simulink library "microgridLibrary"  (R2019b)
settings: Solver=VariableStepAuto  StartTime=0.0  StopTime=10.0  RelTol=1e-3
undefined symbols (not defined in the file or in its folder): Aa, BR, D1, Delta, DiscIntNeverNeededParam, Fn, gcbh, Ion, kv, Lithium, Ls, Pa, Pb, Pc, Rs, sps_rtmsupport, StationData, Ts, Ts_Control, Vn, Vnom
libraries: powerlib x80, simulink x29, powerlib_meascontrol x28, sps_avr x5, spsDieselMotorModel x3, electricdrivelib x2, re_lib x1
(part 3 of 6)

== system microgridLibrary/Diesel Generator (GOV, AVR only)/Selected Measurements ==
  m : Inport
  Bus Creator : BusCreator  Inputs=7
  Bus Selector : BusSelector  OutputSignals="Mechanical.Electrical power  Pe (pu),Mechanical.Rotor speed  wm  (pu),Output active power   Peo (pu),Output reactive power  Qeo (pu)"
  to W : Gain  Gain=Pn
  to W1 : Gain  Gain=Pn
  to W2 : Gain  Gain=Pn
  sm : Outport  VectorParamsAs1DForOutWhenUnconnected=off
  wires:
  to W2/1 -> Bus Creator/7  "Reactive Power (W)"
  to W1/1 -> Bus Creator/6  "Active Power (W)"
  Bus Selector/2 -> Bus Creator/3  "<Rotor speed  wm  (pu)>"
  Bus Creator/1 -> sm/1
  to W/1 -> Bus Creator/1  "Electrical Power (W)"
  Bus Selector/3 -> Bus Creator/4, to W1/1  "<Output active power   Peo (pu)>"
  Bus Selector/1 -> to W/1, Bus Creator/2  "<Electrical power  Pe (pu)>"
  Bus Selector/4 -> Bus Creator/5, to W2/1  "<Output reactive power  Qeo (pu)>"
  m/1 -> Bus Selector/1

== system microgridLibrary/Diesel Generator (Simple Controls)/Continuous ==
  wref (pu) : Inport
  Vref (pu) : Inport  Port=2
  Diesel Engine Governor : spsDieselMotorModel/Diesel Engine Governor  K=29  Tr=[0.01 0.02 0.2]  Ta=[0.25 0.009 0.0384]  Tlim=[0 1.1]  Td=0.024  Pm0=0.84379
      settings: SourceProductName=Simscape Electrical  SourceProductBaseCode=PS
  Excitation System : sps_avr/AC1A Excitation System  Tr=20e-3  KaTa=[400 0.02]  VAminmax=[-14.5 14.5]  VRminmax=[-5.43 6.03]  KfTf=[0.03 1.0]  TbTc=[0 0]  KeTe=[1.0 0.80]  Ve12=[4.18 3.14]  SeVe12=[0.10 0.03]  Kd=0.38  Kc=0.20  v0=[1 1.3376]  TsBlock=0
      settings: SourceProductName=Simscape Electrical  SourceProductBaseCode=PS
  Generator Measures : Subsystem
  Ground : Ground
  Selected Measurements : Subsystem
  Shunt : powerlib/Elements/Three-Phase Parallel RLC Load  LConnTagsString=A|B|C  Configuration=Y (grounded)  NominalVoltage=Vn  Vabc=[1e3 1e3 1e3]  Vabcp=[1e3 1e3 1e3]  NominalFrequency=Fn  UnbalancedPower=off  ActivePower=Pn*0.05  InductivePower=0  CapacitivePower=0  Pabc=[10e3 9e3 11e3]  QLabc=[100 90 110]  QCabc=[100 90 110]  Pabcp=[10e3 9e3 11e3]  QLabcp=[100 90 110]  QCabcp=[100 90 110]  Measurements=None  LoadType=constant Z
      settings: SourceProductName=Simscape Electrical
  Synchronous Machine : powerlib/Machines/Synchronous Machine pu Standard  PresetModel=No  MechanicalLoad=Mechanical power Pm  ShowDetailedParameters=on  RotorType=Salient-pole  Units=per unit standard parameters  MeasurementBus=off  NominalParameters=[ Pn Vn Fn]  Reactances1=[ 1.81, 0.3, 0.23, 1.76, 0.65, 0.25, 0.15 ]  Reactances2="[ 1.305, 0.296, 0.252, 0.474,  0.243,  0.18 ]"  dAxisTimeConstants=Open-circuit  qAxisTimeConstants=Short-circuit  TimeConstants1="[ 4.4849  0.0681  0.1  ]"  TimeConstants2=[ 8.0, 0.03, 1.0, 0.07 ]  TimeConstants3="[  4.49  0.0681  0.0513  ]"  TimeConstants4=[ 8.0, 0.03, 0.3371, 0.0295 ]  TimeConstants5=[ 1.01, 0.053, 0.1 ]  TimeConstants6=[ 1.3201, 0.023, 1.0, 0.07 ]  TimeConstants7=[0.012 0.003 0.003]  TimeConstants8=[ 1.3201, 0.0231, 0.3371, 0.0295 ]  StatorResistance=0.003  Mechanical=[3.7 0 1 ]  PolePairs=20  InitialConditions=[0 -68.3001 0.841667 0.841667 0.841667 4.44859e-14 -120 120 1.3376]  SetSaturation=off  Saturation=[0.6404,0.7127,0.8441,0.9214,0.9956,1.082,1.19,1.316,1.457;0.7,0.7698,0.8872,0.9466,0.9969,1.046,1.1,1.151,1.201]  LoadFlowParameters=[1,0,0,0,0]  TsPowergui=0  TsBlock=-1  IterativeModel=Trapezoidal non iterative  IterativeDiscreteModel=Trapezoidal non iterative  BusType=swing  Pref=Pn*P0  Qref=0  Qmin=-inf  Qmax=inf  PLF=0  QLF=0
      settings: SourceProductName=Simscape Electrical
  A : PMIOPort  Side=Right
  B : PMIOPort  Port=2  Side=Right
  C : PMIOPort  Port=3  Side=Right
  m : Outport  VectorParamsAs1DForOutWhenUnconnected=off
  wires:
  Generator Measures/3(wm) -> Diesel Engine Governor/2
  Vref (pu)/1 -> Excitation System/1
  Selected Measurements/1(sm) -> m/1
  Synchronous Machine/1 -> Generator Measures/1(m), Selected Measurements/1(m)
  Ground/1 -> Excitation System/4
  Generator Measures/1(Ifd) -> Excitation System/3
  Diesel Engine Governor/1 -> Synchronous Machine/1
  wref (pu)/1 -> Diesel Engine Governor/1
  Excitation System/1 -> Synchronous Machine/2
  Generator Measures/2(Vt) -> Excitation System/2
  connections:
  Synchronous Machine/RConn1 -- Shunt/LConn1 -- A/RConn1
  Synchronous Machine/RConn3 -- Shunt/LConn3 -- C/RConn1
  Synchronous Machine/RConn2 -- Shunt/LConn2 -- B/RConn1

== system microgridLibrary/Diesel Generator (Simple Controls)/Discrete ==
  wref (pu) : Inport
  Vref (pu) : Inport  Port=2
  Diesel Engine Governor : Subsystem  mask(Diesel Engine & Governor){K=29, Tr=[0.01 0.02 0.2], Ta=[0.25 0.009 0.0384], Tlim=[0 1.1], Td=0.024, Pm0=0.84379, Ts=Ts}
      mask prompts: K "Regulator gain K:"; Tr "Regulator time constants [T1 T2 T3 ] (s) :"; Ta "Actuator time constants [T4 T5 T6] (s) :"; Tlim "Torque limits [Tmin Tmax] (pu) :"; Td "Engine time delay Td (s) :"; Pm0 "Initial value of mechanical power  Pm0 (pu) :"; Ts "Sample Time (s)"
      mask help:
      | This block implements a diesel engine and governor system:
      | 1st and 2nd inputs: Desired and actual speed (pu)
      | Output: Diesel engine mechanical power.Motor inertia should be combined with generator.
      | Controller transfer function:
      |      Hc=K.(1+T3.s)/(1+T1.s+T1.T2.s^2)
      | Actuator transfer function :
      |      Ha= (1+T4.s) / [ (s (1+T5.s)(1+T6.s) ]
      | Motor :
      |      Time delay Td
      |
      | (See reference in Tutorial Session 5)
  Excitation System : sps_avr/AC1A Excitation System  Tr=20e-3  KaTa=[400 0.02]  VAminmax=[-14.5 14.5]  VRminmax=[-5.43 6.03]  KfTf=[0.03 1.0]  TbTc=[0 0]  KeTe=[1.0 0.80]  Ve12=[4.18 3.14]  SeVe12=[0.10 0.03]  Kd=0.38  Kc=0.20  v0=[1 1.3376]  TsBlock=Ts
      settings: SourceProductName=Simscape Electrical  SourceProductBaseCode=PS
  Generator Measures : Subsystem
  Ground : Ground
  Selected Measurements : Subsystem
  Shunt : powerlib/Elements/Three-Phase Parallel RLC Load  LConnTagsString=A|B|C  Configuration=Y (grounded)  NominalVoltage=Vn  Vabc=[1e3 1e3 1e3]  Vabcp=[1e3 1e3 1e3]  NominalFrequency=Fn  UnbalancedPower=off  ActivePower=Pn*0.05  InductivePower=0  CapacitivePower=0  Pabc=[10e3 9e3 11e3]  QLabc=[100 90 110]  QCabc=[100 90 110]  Pabcp=[10e3 9e3 11e3]  QLabcp=[100 90 110]  QCabcp=[100 90 110]  Measurements=None  LoadType=constant Z
      settings: SourceProductName=Simscape Electrical
  Synchronous Machine : powerlib/Machines/Synchronous Machine pu Standard  PresetModel=No  MechanicalLoad=Mechanical power Pm  ShowDetailedParameters=on  RotorType=Salient-pole  Units=per unit standard parameters  MeasurementBus=off  NominalParameters=[ Pn Vn Fn]  Reactances1=[ 1.81, 0.3, 0.23, 1.76, 0.65, 0.25, 0.15 ]  Reactances2="[ 1.305, 0.296, 0.252, 0.474,  0.243,  0.18 ]"  dAxisTimeConstants=Open-circuit  qAxisTimeConstants=Short-circuit  TimeConstants1="[ 4.4849  0.0681  0.1  ]"  TimeConstants2=[ 8.0, 0.03, 1.0, 0.07 ]  TimeConstants3="[  4.49  0.0681  0.0513  ]"  TimeConstants4=[ 8.0, 0.03, 0.3371, 0.0295 ]  TimeConstants5=[ 1.01, 0.053, 0.1 ]  TimeConstants6=[ 1.3201, 0.023, 1.0, 0.07 ]  TimeConstants7=[0.012 0.003 0.003]  TimeConstants8=[ 1.3201, 0.0231, 0.3371, 0.0295 ]  StatorResistance=0.003  Mechanical=[3.7 0 1 ]  PolePairs=20  InitialConditions=[0 -68.3001 0.841667 0.841667 0.841667 4.44859e-14 -120 120 1.3376]  SetSaturation=off  Saturation=[0.6404,0.7127,0.8441,0.9214,0.9956,1.082,1.19,1.316,1.457;0.7,0.7698,0.8872,0.9466,0.9969,1.046,1.1,1.151,1.201]  LoadFlowParameters=[1,0,0,0,0]  TsPowergui=0  TsBlock=Ts  IterativeModel=Trapezoidal non iterative  IterativeDiscreteModel=Trapezoidal non iterative  BusType=PQ  Pref=Pn*P0  Qref=0  Qmin=-inf  Qmax=inf  PLF=0  QLF=0
      settings: SourceProductName=Simscape Electrical
  A : PMIOPort  Side=Right
  B : PMIOPort  Port=2  Side=Right
  C : PMIOPort  Port=3  Side=Right
  m : Outport  VectorParamsAs1DForOutWhenUnconnected=off
  wires:
  Excitation System/1 -> Synchronous Machine/2
  wref (pu)/1 -> Diesel Engine Governor/1(wref (pu))
  Diesel Engine Governor/1(Pmec (pu)) -> Synchronous Machine/1
  Generator Measures/1(Ifd) -> Excitation System/3
  Ground/1 -> Excitation System/4
  Synchronous Machine/1 -> Selected Measurements/1(m), Generator Measures/1(m)
  Selected Measurements/1(sm) -> m/1
  Generator Measures/2(Vt) -> Excitation System/2
  Vref (pu)/1 -> Excitation System/1
  Generator Measures/3(wm) -> Diesel Engine Governor/2(w (pu))
  connections:
  Synchronous Machine/RConn2 -- Shunt/LConn2 -- B/RConn1
  Synchronous Machine/RConn3 -- Shunt/LConn3 -- C/RConn1
  Synchronous Machine/RConn1 -- Shunt/LConn1 -- A/RConn1

== system microgridLibrary/Energy Storage (PQ Model)/Charge Limits ==
  SOC (%) : Inport
  Pin : Inport  Port=2
  Qin : Inport  Port=3
  Overcharge Check : Subsystem
  Undercharge Check : Subsystem
  Pbatt : Outport  VectorParamsAs1DForOutWhenUnconnected=off
  Qbatt : Outport  Port=2  VectorParamsAs1DForOutWhenUnconnected=off
  wires:
  SOC (%)/1 -> Overcharge Check/1(SOC (%)), Undercharge Check/1(SOC (%))
  Undercharge Check/2(Qout) -> Qbatt/1
  Pin/1 -> Overcharge Check/2(Pin)
  Overcharge Check/1(Pout) -> Undercharge Check/2(Pin)
  Qin/1 -> Overcharge Check/3(Qin)
  Undercharge Check/1(Pout) -> Pbatt/1  "Pbatt"
  Overcharge Check/2(Qout) -> Undercharge Check/3(Qin)

== system microgridLibrary/Energy Storage (PQ Model)/Disable PQ Source if VF Control ==
  Pdes : Inport
  Mode : Inport  Port=2
  Qdes : Inport  Port=3
  Constant : Constant  Value=0
  Constant1 : Constant  Value=0
  Switch2 : Switch  Criteria=u2 > Threshold
  Switch3 : Switch  Criteria=u2 > Threshold
  Pbatt : Outport  VectorParamsAs1DForOutWhenUnconnected=off
  Qbatt : Outport  Port=2  VectorParamsAs1DForOutWhenUnconnected=off
  wires:
  Mode/1 -> Switch3/2, Switch2/2
  Pdes/1 -> Switch2/1
  Switch2/1 -> Pbatt/1
  Constant1/1 -> Switch3/3
  Switch3/1 -> Qbatt/1
  Constant/1 -> Switch2/3
  Qdes/1 -> Switch3/1

== system microgridLibrary/Energy Storage (PQ Model)/Power Measures ==
  EMT : Subsystem  VariantControl=EMT
  Phasor : Subsystem  VariantControl=Phasor
  A : PMIOPort  Side=Left
  a : PMIOPort  Port=2  Side=Right
  B : PMIOPort  Port=3  Side=Left
  b : PMIOPort  Port=4  Side=Right
  C : PMIOPort  Port=5  Side=Left
  c : PMIOPort  Port=6  Side=Right
  P : Outport  VectorParamsAs1DForOutWhenUnconnected=off
  Q : Outport  Port=2  VectorParamsAs1DForOutWhenUnconnected=off

== system microgridLibrary/Energy Storage (PQ Model)/Reactive Power Capability ==
  Pin : Inport
  Qin : Inport  Port=2
  Constant : Constant  Value=Pnom
  Math Function : Math  Operator=square  SaturateOnIntegerOverflow=on
  Math Function1 : Math  Operator=square  SaturateOnIntegerOverflow=on
  Saturation Dynamic : simulink/Discontinuities/Saturation Dynamic  OutMin=[]  OutMax=[]  OutDataTypeStr=Inherit: Same as second input  OutDataType=fixdt(1, 16)  OutScaling=2^-10  DoSatur=off
  Sqrt : Sqrt  SaturateOnIntegerOverflow=on
  Sum : Sum  Inputs=-+|
  Unary Minus : UnaryMinus
  Qout : Outport  VectorParamsAs1DForOutWhenUnconnected=off
  wires:
  Sqrt/1 -> Saturation Dynamic/1, Unary Minus/1
  Math Function1/1 -> Sum/1
  Math Function/1 -> Sum/2
  Constant/1 -> Math Function/1
  Sum/1 -> Sqrt/1
  Unary Minus/1 -> Saturation Dynamic/3
  Saturation Dynamic/1 -> Qout/1
  Pin/1 -> Math Function1/1
  Qin/1 -> Saturation Dynamic/2

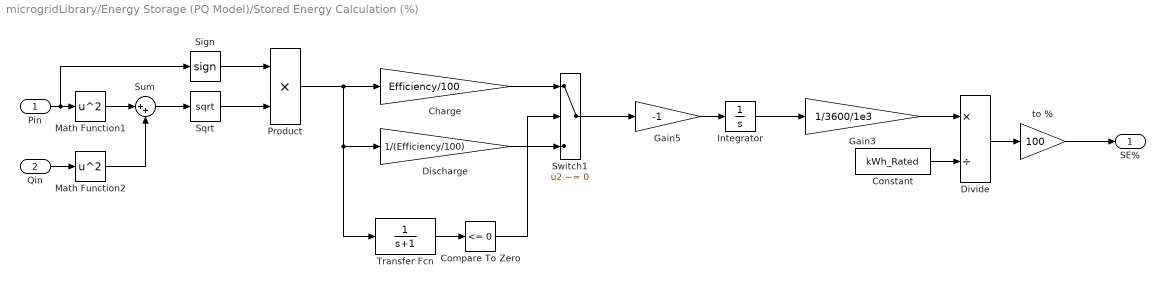
== system microgridLibrary/Energy Storage (PQ Model)/Stored Energy Calculation (%) ==
  Pin : Inport
  Qin : Inport  Port=2
  Charge : Gain  Gain=Efficiency/100
  Compare To Zero : simulink/Logic and Bit Operations/Compare To Zero  relop=<=  OutDataTypeStr=boolean
  Constant : Constant  Value=kWh_Rated
  Discharge : Gain  Gain=1/(Efficiency/100)
  Divide : Product  Inputs=*/
  Gain3 : Gain  Gain=1/3600/1e3
  Gain5 : Gain  Gain=-1
  Integrator : Integrator  InitialCondition=(Initial_kWh_pc/100)*kWh_Rated*3600*1e3
  Math Function1 : Math  Operator=square  SaturateOnIntegerOverflow=on
  Math Function2 : Math  Operator=square  SaturateOnIntegerOverflow=on
  Product : Product
  Sign : Signum
  Sqrt : Sqrt  SaturateOnIntegerOverflow=on
  Sum : Sum  Inputs=|++
  Switch1 : Switch  Criteria=u2 ~= 0
  Transfer Fcn : TransferFcn  Denominator=[1 1]
  to % : Gain  Gain=100
  SE% : Outport  VectorParamsAs1DForOutWhenUnconnected=off
  wires:
  Sign/1 -> Product/1
  Sqrt/1 -> Product/2
  Sum/1 -> Sqrt/1
  Math Function2/1 -> Sum/2
  Math Function1/1 -> Sum/1
  Qin/1 -> Math Function2/1
  Pin/1 -> Math Function1/1, Sign/1
  Product/1 -> Transfer Fcn/1, Discharge/1, Charge/1
  Discharge/1 -> Switch1/3
  Gain5/1 -> Integrator/1
  to %/1 -> SE%/1
  Transfer Fcn/1 -> Compare To Zero/1
  Switch1/1 -> Gain5/1
  Gain3/1 -> Divide/1
  Constant/1 -> Divide/2
  Charge/1 -> Switch1/1
  Divide/1 -> to %/1
  Compare To Zero/1 -> Switch1/2
  Integrator/1 -> Gain3/1

== system microgridLibrary/Fault /Fault A ==
  c : Inport
  Breaker : PMComponent  PhysicalDomain=powersysdomain  LeftPortType=p1  RightPortType=p1  LConnTagsString=a  RConnTagsString=__new0  mask(InnerPowersysBlock){}
  ITAIL : Terminator
  Model : Subsystem
  1 : PMIOPort  Side=Left
  2 : PMIOPort  Port=2  Side=Right
  tag scope: LibraryTag=global
  wires:
  [LibraryTag] -> ITAIL/1
  Model/1(gate) -> [LibraryTag]
  [LibraryTag] -> Model/2(Uswitch)
  c/1 -> Model/1("gate ")
  connections:
  1/RConn1 -- Breaker/LConn1
  2/RConn1 -- Breaker/RConn1

== system microgridLibrary/Fault /Fault B ==
  c : Inport
  Breaker : PMComponent  PhysicalDomain=powersysdomain  LeftPortType=p1  RightPortType=p1  LConnTagsString=a  RConnTagsString=__new0  mask(InnerPowersysBlock){}
  ITAIL : Terminator
  Model : Subsystem
  1 : PMIOPort  Side=Left
  2 : PMIOPort  Port=2  Side=Right
  tag scope: LibraryTag=global
  wires:
  [LibraryTag] -> ITAIL/1
  Model/1(gate) -> [LibraryTag]
  [LibraryTag] -> Model/2(Uswitch)
  c/1 -> Model/1("gate ")
  connections:
  1/RConn1 -- Breaker/LConn1
  2/RConn1 -- Breaker/RConn1

== system microgridLibrary/Fault /Fault C ==
  c : Inport
  Breaker : PMComponent  PhysicalDomain=powersysdomain  LeftPortType=p1  RightPortType=p1  LConnTagsString=a  RConnTagsString=__new0  mask(InnerPowersysBlock){}
  ITAIL : Terminator
  Model : Subsystem
  1 : PMIOPort  Side=Left
  2 : PMIOPort  Port=2  Side=Right
  tag scope: LibraryTag=global
  wires:
  [LibraryTag] -> ITAIL/1
  Model/1(gate) -> [LibraryTag]
  [LibraryTag] -> Model/2(Uswitch)
  c/1 -> Model/1("gate ")
  connections:
  1/RConn1 -- Breaker/LConn1
  2/RConn1 -- Breaker/RConn1

== system microgridLibrary/Grid Source Phasor Load Flow/Model ==
  Constant : Constant  Value=complex(cos(Pa),sin(Pa))
  Constant1 : Constant  Value=complex(cos(Pb),sin(Pb))
  Constant2 : Constant  Value=complex(cos(Pc),sin(Pc))
  Gain : Gain  Gain=Aa
  Initial Voltage : Subsystem
  Mux : Mux  Inputs=3
  Product : Product
  Out1 : Outport
  wires:
  Constant1/1 -> Mux/2
  Constant/1 -> Mux/1
  Constant2/1 -> Mux/3
  Mux/1 -> Product/1
  Product/1 -> Out1/1
  Initial Voltage/1(Aa) -> Gain/1
  Gain/1 -> Product/2

== system microgridLibrary/Grid-Connected Battery (EMT with Simple Controls)/Battery Controller ==
  m : Inport
  PQref : Inport  Port=2
  Compute PQ : Subsystem
  "P,Q Control " : Subsystem  TreatAsAtomicUnit=on
  to PU : Gain  Gain=1/Pnom
  Idq_ref : Outport  VectorParamsAs1DForOutWhenUnconnected=off
  wires:
  "P,Q Control "/1(Idq_ref) -> Idq_ref/1
  to PU/1 -> "P,Q Control "/1(PQref)
  m/1 -> Compute PQ/1(m)
  PQref/1 -> to PU/1
  Compute PQ/1(PQm) -> "P,Q Control "/2(m)

== system microgridLibrary/Grid-Connected Battery (EMT with Simple Controls)/DC Link ==
  C1 : powerlib/Elements/Series RLC Branch  LConnTagsString=__new0  RConnTagsString=__new0  BranchType=C  Resistance=1.0  Inductance=1.0  SetiL0=off  InitialCurrent=0  Capacitance=Clink  Setx0=on  InitialVoltage=Vnom_dc/2  Measurements=None
      settings: SourceProductName=Simscape Electrical
  C2 : powerlib/Elements/Series RLC Branch  LConnTagsString=__new0  RConnTagsString=__new0  BranchType=C  Resistance=1e5  Inductance=1.0  SetiL0=off  InitialCurrent=0  Capacitance=Clink  Setx0=on  InitialVoltage=Vnom_dc/2  Measurements=None
      settings: SourceProductName=Simscape Electrical
  PV+ : PMIOPort  Side=Left
  PV-- : PMIOPort  Port=2  Side=Left
  Inv+ : PMIOPort  Port=3  Side=Right
  N : PMIOPort  Port=4  Side=Right
  Inv-- : PMIOPort  Port=5  Side=Right
  connections:
  Inv--/RConn1 -- PV--/RConn1 -- C2/RConn1
  C1/RConn1 -- N/RConn1 -- C2/LConn1
  Inv+/RConn1 -- PV+/RConn1 -- C1/LConn1

== system microgridLibrary/Grid-Connected Battery (EMT with Simple Controls)/Grid Inverter ==
  note: Harmonic Filter
  Uref : Inport
  10 kvar : powerlib/Elements/Three-Phase Series RLC Load  LConnTagsString=A|B|C  Configuration=Delta  NominalVoltage=Vnom_sec  Vabc=[1e3 1e3 1e3]  Vabcp=[1e3 1e3 1e3]  NominalFrequency=Fnom  UnbalancedPower=off  ActivePower=Pc  InductivePower=0  CapacitivePower=Qc  Pabc=[10e3 9e3 11e3]  QLabc=[100 90 110]  QCabc=[100 90 110]  Pabcp=[10e3 9e3 11e3]  QLabcp=[100 90 110]  QCabcp=[100 90 110]  Measurements=None  LoadType=constant Z
      settings: SourceProductName=Simscape Electrical
  100 kVA 260V / 25 kV : powerlib/Elements/Three-Phase Transformer (Two Windings)  Winding1Connection=Yg  Winding2Connection=Delta (D1)  CoreType=Three single-phase transformers  SetSaturation=off  Hysteresis=off  DataFile='hysteresis'  SetInitialFlux=off  Measurements=None  UNITS=pu  NominalPower=[Pnom Fnom ]  Winding1=[ Vnom_prim , Rxf/2 , Lxf/2 ]  Winding2=[ Vnom_sec , Rxf/2 , Lxf/2 ]  Rm=200  Lm=200  L0=0.5  Saturation=[ 0,0 ; 0.0024,1.2 ; 1.0,1.52 ]  InitialFluxes=[ 0.8 , -0.8 , 0.7 ]  BreakLoop=off  DiscreteSolver=Trapezoidal iterative  DataType=off  TransfoNumber=0
      settings: SourceProductName=Simscape Electrical
  B1 : powerlib/Measurements/Three-Phase V-I Measurement  VoltageMeasurement=phase-to-ground  SetLabelV=off  LabelV=Vabc_B1  Vpu=off  VpuLL=off  CurrentMeasurement=yes  SetLabelI=off  LabelI=Iabc_B1  Ipu=off  Pbase=100e6  Vbase=500e3  OutputType=Magnitude  PhasorSimulation=off  PSBequivalent=0
      settings: SourceProductName=Simscape Electrical
  Bus Creator : BusCreator  Inputs=2
  Ground : Ground
  L : powerlib/Elements/Three-Phase Series RLC Branch  LConnTagsString=A|B|C  RConnTagsString=A|B|C  BranchType=RL  Resistance=Rchoke*Zbase  Inductance=Lchoke*Zbase/(2*pi*Fnom)  Capacitance=inf  Measurements=None
      settings: SourceProductName=Simscape Electrical
  Three-Level NPC Converter : powerlib/Power Electronics/Three-Level NPC Converter  ModelType=Average model (Uref-controlled)  Ron=1e-3  Rs=1e6  Cs=inf  Vforward=[0,0]  Ron_Diode=1e-3  Rs_Diode=1e6  Cs_Diode=inf  Vf_Diode=1e-3  Rs_CurrentSource=inf
      settings: SourceProductName=Simscape Electrical  SourceProductBaseCode=PS
  Inv+ : PMIOPort  Side=Left
  N : PMIOPort  Port=2  Side=Left
  Inv-- : PMIOPort  Port=3  Side=Left
  A : PMIOPort  Port=4  Side=Right
  B : PMIOPort  Port=5  Side=Right
  C : PMIOPort  Port=6  Side=Right
  m : Outport  VectorParamsAs1DForOutWhenUnconnected=off
  wires:
  Uref/1 -> Three-Level NPC Converter/1
  B1/1 -> Bus Creator/1  "Vabc"
  B1/2 -> Bus Creator/2  "Iabc"
  Bus Creator/1 -> m/1
  Ground/1 -> Three-Level NPC Converter/2
  connections:
  B1/RConn3 -- C/RConn1
  B1/RConn2 -- B/RConn1
  B1/RConn1 -- A/RConn1
  10 kvar/LConn1 -- 100 kVA 260V / 25 kV/RConn1 -- L/RConn1
  Three-Level NPC Converter/RConn1 -- Inv+/RConn1
  Three-Level NPC Converter/RConn3 -- Inv--/RConn1
  L/RConn3 -- 100 kVA 260V / 25 kV/RConn3 -- 10 kvar/LConn3
  L/RConn2 -- 100 kVA 260V / 25 kV/RConn2 -- 10 kvar/LConn2
  100 kVA 260V / 25 kV/LConn3 -- B1/LConn3
  100 kVA 260V / 25 kV/LConn2 -- B1/LConn2
  100 kVA 260V / 25 kV/LConn1 -- B1/LConn1
  Three-Level NPC Converter/LConn1 -- L/LConn1
  Three-Level NPC Converter/LConn2 -- L/LConn2
  Three-Level NPC Converter/LConn3 -- L/LConn3
  N/RConn1 -- Three-Level NPC Converter/RConn2

== system microgridLibrary/Grid-Connected Battery (EMT with Simple Controls)/Inverter Control ==
  Vabc_prim : Inport  PortDimensions=3
  Iabc_prim : Inport  Port=2  PortDimensions=3
  Idq_ref : Inport  Port=3
  Current Control : Subsystem  TreatAsAtomicUnit=on
  Overmodulation : powerlib_meascontrol/Pulse & Signal Generators/Overmodulation  OverModType=Flat top
      settings: SourceProductName=Simscape Electrical  SourceProductBaseCode=PS
  PLL & Measurements : Subsystem
  Unit Delay : UnitDelay  SampleTime=Ts_Control  HasFrameUpgradeWarning=on
  Uref : Outport  VectorParamsAs1DForOutWhenUnconnected=off
  wires:
  Unit Delay/1 -> Overmodulation/1
  Overmodulation/1 -> Uref/1
  Current Control/1(Uabc) -> Unit Delay/1
  Idq_ref/1 -> Current Control/4(IdIq_ref)
  PLL & Measurements/1(wt) -> Current Control/1(wt)
  PLL & Measurements/2(VdVq_prim) -> Current Control/2(VdVq_meas)
  PLL & Measurements/3(IdIq_prim) -> Current Control/3(IdIq_meas)
  Iabc_prim/1 -> PLL & Measurements/2(Iabc_prim)
  Vabc_prim/1 -> PLL & Measurements/1(Vabc_prim)

== system microgridLibrary/Grid-Connected Battery (EMT with Simple Controls)/Measures ==
  Grid : Inport
  Battery : Inport  Port=2
  Bus Creator : BusCreator  Inputs=2
  Bus Creator1 : BusCreator  Inputs=4
  Bus Selector2 : BusSelector  OutputSignals=Vabc,Iabc
  "Power (3ph, Instantaneous)" : powerlib_meascontrol/Measurements/Power (3ph, Instantaneous)
      settings: SourceProductName=Simscape Electrical
  m : Outport  VectorParamsAs1DForOutWhenUnconnected=off
  wires:
  Bus Creator1/1 -> Bus Creator/1  "Grid"
  "Power (3ph, Instantaneous)"/2 -> Bus Creator1/4  "Q"
  Grid/1 -> Bus Selector2/1
  Battery/1 -> Bus Creator/2  "Battery"
  Bus Creator/1 -> m/1
  "Power (3ph, Instantaneous)"/1 -> Bus Creator1/3  "P"
  Bus Selector2/2 -> Bus Creator1/2, "Power (3ph, Instantaneous)"/2  "<Iabc>"
  Bus Selector2/1 -> Bus Creator1/1, "Power (3ph, Instantaneous)"/1  "<Vabc>"

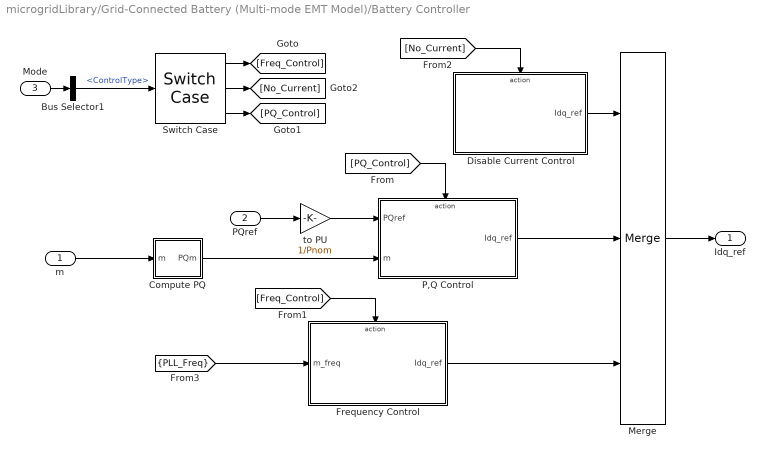
== system microgridLibrary/Grid-Connected Battery (Multi-mode EMT Model)/Battery Controller ==
  m : Inport
  PQref : Inport  Port=2
  Mode : Inport  Port=3  SampleTime=Ts_Control
  Bus Selector1 : BusSelector  OutputSignals=ControlType
  Compute PQ : Subsystem
  Disable Current Control : Subsystem  TreatAsAtomicUnit=on
  "Frequency Control " : Subsystem  TreatAsAtomicUnit=on
  Merge : Merge  Inputs=3
  "P,Q Control " : Subsystem  TreatAsAtomicUnit=on
  Switch Case : SwitchCase  CaseConditions={1,2}
  to PU : Gain  Gain=1/Pnom
  Idq_ref : Outport  VectorParamsAs1DForOutWhenUnconnected=off
  wires:
  Merge/1 -> Idq_ref/1
  Compute PQ/1(PQm) -> "P,Q Control "/2(m)
  PQref/1 -> to PU/1
  [Freq_Control] -> "Frequency Control "/Action
  m/1 -> Compute PQ/1(m)
  [PQ_Control] -> "P,Q Control "/Action
  Switch Case/3 -> [PQ_Control]
  Switch Case/1 -> [Freq_Control]
  to PU/1 -> "P,Q Control "/1(PQref)
  "Frequency Control "/1(Idq_ref) -> Merge/3
  Mode/1 -> Bus Selector1/1
  Bus Selector1/1 -> Switch Case/1  "<ControlType>"
  Switch Case/2 -> [No_Current]
  [No_Current] -> Disable Current Control/Action
  "P,Q Control "/1(Idq_ref) -> Merge/2
  Disable Current Control/1(Idq_ref) -> Merge/1
  [PLL_Freq] -> "Frequency Control "/1(m_freq)

== system microgridLibrary/Grid-Connected Battery (Multi-mode EMT Model)/DC Link ==
  C1 : powerlib/Elements/Series RLC Branch  LConnTagsString=__new0  RConnTagsString=__new0  BranchType=C  Resistance=1.0  Inductance=1.0  SetiL0=off  InitialCurrent=0  Capacitance=Clink  Setx0=on  InitialVoltage=Vnom_dc/2  Measurements=None
      settings: SourceProductName=Simscape Electrical
  C2 : powerlib/Elements/Series RLC Branch  LConnTagsString=__new0  RConnTagsString=__new0  BranchType=C  Resistance=1e5  Inductance=1.0  SetiL0=off  InitialCurrent=0  Capacitance=Clink  Setx0=on  InitialVoltage=Vnom_dc/2  Measurements=None
      settings: SourceProductName=Simscape Electrical
  PV+ : PMIOPort  Side=Left
  PV-- : PMIOPort  Port=2  Side=Left
  Inv+ : PMIOPort  Port=3  Side=Right
  N : PMIOPort  Port=4  Side=Right
  Inv-- : PMIOPort  Port=5  Side=Right
  connections:
  C1/LConn1 -- PV+/RConn1 -- Inv+/RConn1
  C2/LConn1 -- N/RConn1 -- C1/RConn1
  C2/RConn1 -- PV--/RConn1 -- Inv--/RConn1

== system microgridLibrary/Grid-Connected Battery (Multi-mode EMT Model)/Grid Inverter ==
  note: Harmonic Filter
  Uref : Inport
  10 kvar : powerlib/Elements/Three-Phase Series RLC Load  LConnTagsString=A|B|C  Configuration=Delta  NominalVoltage=Vnom_sec  Vabc=[1e3 1e3 1e3]  Vabcp=[1e3 1e3 1e3]  NominalFrequency=Fnom  UnbalancedPower=off  ActivePower=Pc  InductivePower=0  CapacitivePower=Qc  Pabc=[10e3 9e3 11e3]  QLabc=[100 90 110]  QCabc=[100 90 110]  Pabcp=[10e3 9e3 11e3]  QLabcp=[100 90 110]  QCabcp=[100 90 110]  Measurements=None  LoadType=constant Z
      settings: SourceProductName=Simscape Electrical
  100 kVA 260V / 25 kV : powerlib/Elements/Three-Phase Transformer (Two Windings)  Winding1Connection=Yg  Winding2Connection=Delta (D1)  CoreType=Three single-phase transformers  SetSaturation=off  Hysteresis=off  DataFile='hysteresis'  SetInitialFlux=off  Measurements=None  UNITS=pu  NominalPower=[Pnom Fnom ]  Winding1=[ Vnom_prim , Rxf/2 , Lxf/2 ]  Winding2=[ Vnom_sec , Rxf/2 , Lxf/2 ]  Rm=200  Lm=200  L0=0.5  Saturation=[ 0,0 ; 0.0024,1.2 ; 1.0,1.52 ]  InitialFluxes=[ 0.8 , -0.8 , 0.7 ]  BreakLoop=off  DiscreteSolver=Trapezoidal iterative  DataType=off  TransfoNumber=0
      settings: SourceProductName=Simscape Electrical
  B1 : powerlib/Measurements/Three-Phase V-I Measurement  VoltageMeasurement=phase-to-ground  SetLabelV=off  LabelV=Vabc_B1  Vpu=off  VpuLL=off  CurrentMeasurement=yes  SetLabelI=off  LabelI=Iabc_B1  Ipu=off  Pbase=100e6  Vbase=500e3  OutputType=Magnitude  PhasorSimulation=off  PSBequivalent=0
      settings: SourceProductName=Simscape Electrical
  Bus Creator : BusCreator  Inputs=2
  Ground : Ground
  L : powerlib/Elements/Three-Phase Series RLC Branch  LConnTagsString=A|B|C  RConnTagsString=A|B|C  BranchType=RL  Resistance=Rchoke*Zbase  Inductance=Lchoke*Zbase/(2*pi*Fnom)  Capacitance=inf  Measurements=None
      settings: SourceProductName=Simscape Electrical
  Three-Level NPC Converter : powerlib/Power Electronics/Three-Level NPC Converter  ModelType=Average model (Uref-controlled)  Ron=1e-3  Rs=1e6  Cs=inf  Vforward=[0,0]  Ron_Diode=1e-3  Rs_Diode=1e6  Cs_Diode=inf  Vf_Diode=1e-3  Rs_CurrentSource=inf
      settings: SourceProductName=Simscape Electrical  SourceProductBaseCode=PS
  Inv+ : PMIOPort  Side=Left
  N : PMIOPort  Port=2  Side=Left
  Inv-- : PMIOPort  Port=3  Side=Left
  A : PMIOPort  Port=4  Side=Right
  B : PMIOPort  Port=5  Side=Right
  C : PMIOPort  Port=6  Side=Right
  m : Outport  VectorParamsAs1DForOutWhenUnconnected=off
  wires:
  Ground/1 -> Three-Level NPC Converter/2
  Bus Creator/1 -> m/1
  B1/2 -> Bus Creator/2  "Iabc"
  B1/1 -> Bus Creator/1  "Vabc"
  Uref/1 -> Three-Level NPC Converter/1
  connections:
  N/RConn1 -- Three-Level NPC Converter/RConn2
  Three-Level NPC Converter/LConn3 -- L/LConn3
  Three-Level NPC Converter/LConn2 -- L/LConn2
  Three-Level NPC Converter/LConn1 -- L/LConn1
  100 kVA 260V / 25 kV/LConn1 -- B1/LConn1
  100 kVA 260V / 25 kV/LConn2 -- B1/LConn2
  100 kVA 260V / 25 kV/LConn3 -- B1/LConn3
  10 kvar/LConn2 -- 100 kVA 260V / 25 kV/RConn2 -- L/RConn2
  10 kvar/LConn3 -- 100 kVA 260V / 25 kV/RConn3 -- L/RConn3
  Three-Level NPC Converter/RConn3 -- Inv--/RConn1
  Three-Level NPC Converter/RConn1 -- Inv+/RConn1
  L/RConn1 -- 100 kVA 260V / 25 kV/RConn1 -- 10 kvar/LConn1
  B1/RConn1 -- A/RConn1
  B1/RConn2 -- B/RConn1
  B1/RConn3 -- C/RConn1

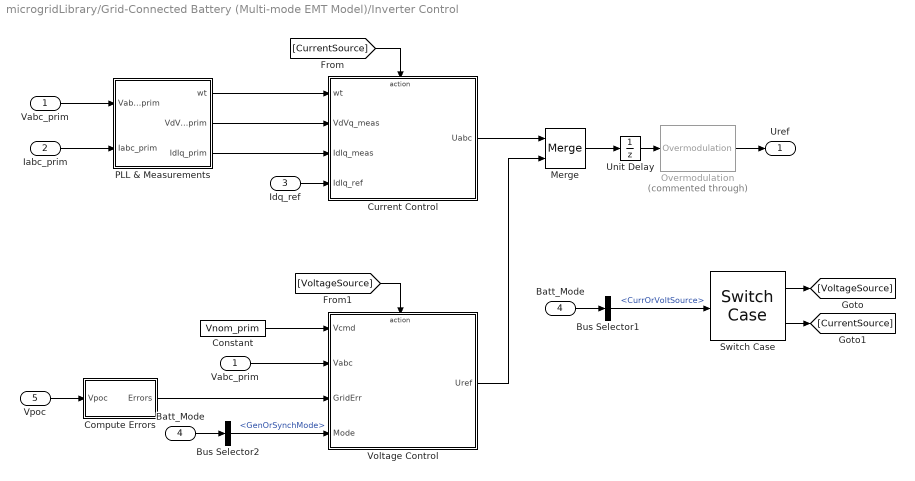
== system microgridLibrary/Grid-Connected Battery (Multi-mode EMT Model)/Inverter Control ==
  Vabc_prim : Inport  PortDimensions=3
  Iabc_prim : Inport  Port=2  PortDimensions=3
  Idq_ref : Inport  Port=3
  Batt_Mode : Inport  Port=4  PortDimensions=1  SampleTime=Ts_Control
  Vpoc : Inport  Port=5
  "Batt_Mode " : InportShadow  Port=4  PortDimensions=1  SampleTime=Ts_Control
  Bus Selector1 : BusSelector  OutputSignals=Batt_Mode.CurrOrVoltSource
  Bus Selector2 : BusSelector  OutputSignals=Batt_Mode.GenOrSynchMode
  Compute Errors : Subsystem
  Constant : Constant  Value=Vnom_prim
  Current Control : Subsystem  TreatAsAtomicUnit=on
  Merge : Merge
  Overmodulation : powerlib_meascontrol/Pulse & Signal Generators/Overmodulation  Commented=through  OverModType=Flat top
      settings: SourceProductName=Simscape Electrical  SourceProductBaseCode=PS
  PLL & Measurements : Subsystem
  Switch Case : SwitchCase
  Unit Delay : UnitDelay  SampleTime=Ts_Control  HasFrameUpgradeWarning=on
  "Vabc_prim " : InportShadow  PortDimensions=3
  Voltage Control : Subsystem  TreatAsAtomicUnit=on
  Uref : Outport  VectorParamsAs1DForOutWhenUnconnected=off
  wires:
  Switch Case/2 -> [CurrentSource]
  Switch Case/1 -> [VoltageSource]
  [CurrentSource] -> Current Control/Action
  [VoltageSource] -> Voltage Control/Action
  Vabc_prim/1 -> PLL & Measurements/1(Vabc_prim)
  Iabc_prim/1 -> PLL & Measurements/2(Iabc_prim)
  PLL & Measurements/3(IdIq_prim) -> Current Control/3(IdIq_meas)
  PLL & Measurements/2(VdVq_prim) -> Current Control/2(VdVq_meas)
  PLL & Measurements/1(wt) -> Current Control/1(wt)
  Idq_ref/1 -> Current Control/4(IdIq_ref)
  Current Control/1(Uabc) -> Merge/1
  Voltage Control/1(Uref) -> Merge/2
  Merge/1 -> Unit Delay/1
  Constant/1 -> Voltage Control/1(Vcmd)
  "Vabc_prim "/1 -> Voltage Control/2(Vabc)
  Overmodulation/1 -> Uref/1
  Unit Delay/1 -> Overmodulation/1
  Batt_Mode/1 -> Bus Selector1/1
  Vpoc/1 -> Compute Errors/1(Vpoc)
  Compute Errors/1(Errors) -> Voltage Control/3(GridErr)
  Bus Selector1/1 -> Switch Case/1  "<CurrOrVoltSource>"
  Bus Selector2/1 -> Voltage Control/4(Mode)  "<GenOrSynchMode>"
  "Batt_Mode "/1 -> Bus Selector2/1

== system microgridLibrary/Grid-Connected Battery (Multi-mode EMT Model)/Measures ==
  Grid : Inport
  Battery : Inport  Port=2
  Bus Creator : BusCreator  Inputs=2
  Bus Creator1 : BusCreator  Inputs=4
  Bus Selector2 : BusSelector  OutputSignals=Vabc,Iabc
  "Power (3ph, Instantaneous)" : powerlib_meascontrol/Measurements/Power (3ph, Instantaneous)
      settings: SourceProductName=Simscape Electrical
  m : Outport  VectorParamsAs1DForOutWhenUnconnected=off
  wires:
  Bus Selector2/1 -> "Power (3ph, Instantaneous)"/1, Bus Creator1/1  "<Vabc>"
  Bus Selector2/2 -> "Power (3ph, Instantaneous)"/2, Bus Creator1/2  "<Iabc>"
  "Power (3ph, Instantaneous)"/1 -> Bus Creator1/3  "P"
  Bus Creator/1 -> m/1
  Battery/1 -> Bus Creator/2  "Battery"
  Grid/1 -> Bus Selector2/1
  "Power (3ph, Instantaneous)"/2 -> Bus Creator1/4  "Q"
  Bus Creator1/1 -> Bus Creator/1  "Grid"

== system microgridLibrary/Ideal Source/Subsystem ==
  Freq (Hz) : Inport
  Constant1 : Constant
  Gain2 : Gain  Gain=2*pi
  Gain3 : Gain  Gain=2*pi*Frequency
  Sum : Sum  Inputs=|+-
  theta integrator1 : Integrator  InitialCondition=2*pi*Frequency  WrappedStateUpperValue=2*pi*60  WrappedStateLowerValue=0
  theta integrator2 : Integrator  InitialCondition=2*pi*Frequency  WrappedStateUpperValue=2*pi*60  WrappedStateLowerValue=0
  Phase : Outport  VectorParamsAs1DForOutWhenUnconnected=off
  wires:
  Gain2/1 -> theta integrator1/1
  Constant1/1 -> Gain3/1
  theta integrator1/1 -> Sum/1
  Sum/1 -> Phase/1
  theta integrator2/1 -> Sum/2
  Gain3/1 -> theta integrator2/1
  Freq (Hz)/1 -> Gain2/1

== system microgridLibrary/Power Equation Wind Turbine (PQ Model)/Active Power Dynamics ==
  In : Inport
  1/Tp : Gain  Gain=1/Tp
  Integrator : Integrator
  Sum : Sum  Inputs=|+-
  Out : Outport  VectorParamsAs1DForOutWhenUnconnected=off
  wires:
  Integrator/1 -> Out/1, Sum/2
  In/1 -> Sum/1
  1/Tp/1 -> Integrator/1
  Sum/1 -> 1/Tp/1

== system microgridLibrary/Power Equation Wind Turbine (PQ Model)/Reactive Power Dynamics ==
  In : Inport
  1/Tq : Gain  Gain=1/Tq
  Integrator : Integrator
  Sum : Sum  Inputs=|+-
  Out : Outport  VectorParamsAs1DForOutWhenUnconnected=off
  wires:
  Sum/1 -> 1/Tq/1
  1/Tq/1 -> Integrator/1
  In/1 -> Sum/1
  Integrator/1 -> Sum/2, Out/1

== system microgridLibrary/Power Equation Wind Turbine (PQ Model)/Wind Turbine Power Equation ==
  Wind (m/s) : Inport
  Constant : Constant  Value=Pselect
  Cubic Power with Cutoff : Subsystem
  Manufacturer Fit : Lookup_n-D  NumberOfTableDimensions=1  BreakpointsForDimension1=Uvec  Table=Pvec  ExtrapMethod=Clip  InternalRulePriority=Speed  RndMeth=Simplest  InputSameDT=on
  Multiport Switch : MultiPortSwitch
  Saturation : Saturate  UpperLimit=inf  LowerLimit=0  ZeroCross=off
      settings: AttributesFormatString=|
      | %<UpperLimit>
      | %<LowerLimit>
  Wind Turbine Properties : Subsystem
  Pwind : Outport  VectorParamsAs1DForOutWhenUnconnected=off
  wires:
  Wind Turbine Properties/1(Pwind) -> Multiport Switch/2
  Manufacturer Fit/1 -> Multiport Switch/4
  Cubic Power with Cutoff/1(Pwind) -> Multiport Switch/3
  Saturation/1 -> Cubic Power with Cutoff/1(Wind (m/s)), Manufacturer Fit/1, Wind Turbine Properties/1(Wind (m/s))
  Constant/1 -> Multiport Switch/1
  Multiport Switch/1 -> Pwind/1
  Wind (m/s)/1 -> Saturation/1

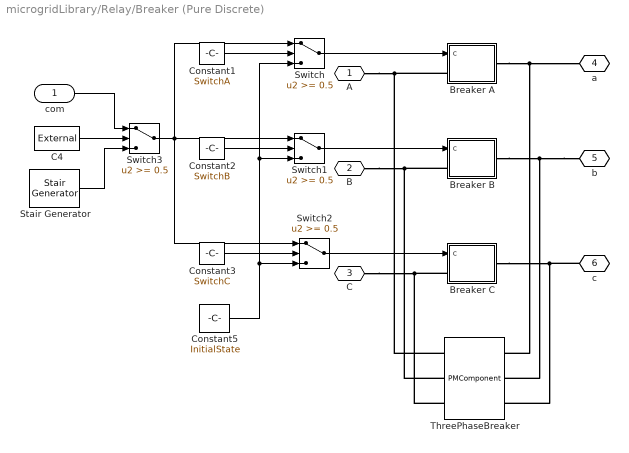
== system microgridLibrary/Relay/Breaker (Pure Discrete) ==
  com : Inport
  Breaker A : Subsystem  DialogController=POWERSYS.PowerSysDialog  LoadFcn=sps_rtmsupport('LoadFcn',gcbh);  StartFcn=sps_rtmsupport('StartFcn',gcbh);  StopFcn=sps_rtmsupport('StopFcn',gcbh);  mask(Breaker){InitialState=InitialState, SwitchingTimes=[ 1/60  5/60 ], External=on, BreakerResistance=BreakerResistance, SnubberResistance=SnubberResistance, SnubberCapacitance=SnubberCapacitance, Measurements=None, MoreParameters=off, NoBreakLoop=off}
      mask prompts: InitialState "Initial status:"; SwitchingTimes "Switching times (s):"; BreakerResistance "Breaker resistance Ron (Ohm):"; SnubberResistance "Snubber resistance Rs (Ohm):"; SnubberCapacitance "Snubber capacitance Cs (F):"; MoreParameters "obsolete"; NoBreakLoop "Enable zero crossing detection (create an algebraic loop)"
      mask help: Implements a circuit breaker. When the external switching time option is selected, a Simulink logical signal is used to control the breaker operation.
      mask init: same as microgridLibrary/Fault /Fault A
      settings: CopyFcn=sps_rtmsupport('CopyFcn',gcbh); powericon('SwitchesCopyFcn','Breaker',gcb)  DeleteFcn=sps_rtmsupport('DeleteFcn',gcbh);  UndoDeleteFcn=sps_rtmsupport('UndoDeleteFcn',gcbh);  ModelCloseFcn=sps_rtmsupport('ModelCloseFcn',gcbh);  PreSaveFcn=sps_rtmsupport('PreSaveFcn',gcbh);  PostSaveFcn=sps_rtmsupport('PostSaveFcn',gcbh);  NameChangeFcn=sps_rtmsupport('NameChangeFcn',gcbh);  PreCopyFcn=sps_rtmsupport('PreCopyFcn',gcbh);  OpenFcn=sps_rtmsupport('OpenFcn',gcbh, [3 7 8 9]);  CloseFcn=sps_rtmsupport('CloseFcn',gcbh);  PreDeleteFcn=sps_rtmsupport('PreDeleteFcn',gcbh);
      mask Help: helpview(psbhelp);
      mask Callback External: powericon('BreakerCback',gcb);
      mask Callback BreakerResistance: powericon('SwitchesEnables',gcb,'Breaker');
      mask TypeOptions Measurements: None | Branch voltage | Branch current | Branch voltage and current
      mask Display: % plot(X.p1,Y.p1,X.p2,Y.p2,X.p3,Y.p3,X.p4,Y.p4,X.p5,Y.p5,X.p6,Y.p6)
  Breaker B : Subsystem  DialogController=POWERSYS.PowerSysDialog  LoadFcn=sps_rtmsupport('LoadFcn',gcbh);  StartFcn=sps_rtmsupport('StartFcn',gcbh);  StopFcn=sps_rtmsupport('StopFcn',gcbh);  mask(Breaker){InitialState=InitialState, SwitchingTimes=[ 1/60  5/60 ], External=on, BreakerResistance=BreakerResistance, SnubberResistance=SnubberResistance, SnubberCapacitance=SnubberCapacitance, Measurements=None, MoreParameters=off, NoBreakLoop=off}
      mask prompts: InitialState "Initial status:"; SwitchingTimes "Switching times (s):"; BreakerResistance "Breaker resistance Ron (Ohm):"; SnubberResistance "Snubber resistance Rs (Ohm):"; SnubberCapacitance "Snubber capacitance Cs (F):"; MoreParameters "obsolete"; NoBreakLoop "Enable zero crossing detection (create an algebraic loop)"
      mask help: Implements a circuit breaker. When the external switching time option is selected, a Simulink logical signal is used to control the breaker operation.
      mask init: same as microgridLibrary/Fault /Fault A
      settings: CopyFcn=sps_rtmsupport('CopyFcn',gcbh); powericon('SwitchesCopyFcn','Breaker',gcb)  DeleteFcn=sps_rtmsupport('DeleteFcn',gcbh);  UndoDeleteFcn=sps_rtmsupport('UndoDeleteFcn',gcbh);  ModelCloseFcn=sps_rtmsupport('ModelCloseFcn',gcbh);  PreSaveFcn=sps_rtmsupport('PreSaveFcn',gcbh);  PostSaveFcn=sps_rtmsupport('PostSaveFcn',gcbh);  NameChangeFcn=sps_rtmsupport('NameChangeFcn',gcbh);  PreCopyFcn=sps_rtmsupport('PreCopyFcn',gcbh);  OpenFcn=sps_rtmsupport('OpenFcn',gcbh, [3 7 8 9]);  CloseFcn=sps_rtmsupport('CloseFcn',gcbh);  PreDeleteFcn=sps_rtmsupport('PreDeleteFcn',gcbh);
      mask Help: helpview(psbhelp);
      mask Callback External: powericon('BreakerCback',gcb);
      mask Callback BreakerResistance: powericon('SwitchesEnables',gcb,'Breaker');
      mask TypeOptions Measurements: None | Branch voltage | Branch current | Branch voltage and current
      mask Display: % plot(X.p1,Y.p1,X.p2,Y.p2,X.p3,Y.p3,X.p4,Y.p4,X.p5,Y.p5,X.p6,Y.p6)
  Breaker C : Subsystem  DialogController=POWERSYS.PowerSysDialog  LoadFcn=sps_rtmsupport('LoadFcn',gcbh);  StartFcn=sps_rtmsupport('StartFcn',gcbh);  StopFcn=sps_rtmsupport('StopFcn',gcbh);  mask(Breaker){InitialState=InitialState, SwitchingTimes=[ 1/60  5/60 ], External=on, BreakerResistance=BreakerResistance, SnubberResistance=SnubberResistance, SnubberCapacitance=SnubberCapacitance, Measurements=None, MoreParameters=off, NoBreakLoop=off}
      mask prompts: InitialState "Initial status:"; SwitchingTimes "Switching times (s):"; BreakerResistance "Breaker resistance Ron (Ohm):"; SnubberResistance "Snubber resistance Rs (Ohm):"; SnubberCapacitance "Snubber capacitance Cs (F):"; MoreParameters "obsolete"; NoBreakLoop "Enable zero crossing detection (create an algebraic loop)"
      mask help: Implements a circuit breaker. When the external switching time option is selected, a Simulink logical signal is used to control the breaker operation.
      mask init: same as microgridLibrary/Fault /Fault A
      settings: CopyFcn=sps_rtmsupport('CopyFcn',gcbh); powericon('SwitchesCopyFcn','Breaker',gcb)  DeleteFcn=sps_rtmsupport('DeleteFcn',gcbh);  UndoDeleteFcn=sps_rtmsupport('UndoDeleteFcn',gcbh);  ModelCloseFcn=sps_rtmsupport('ModelCloseFcn',gcbh);  PreSaveFcn=sps_rtmsupport('PreSaveFcn',gcbh);  PostSaveFcn=sps_rtmsupport('PostSaveFcn',gcbh);  NameChangeFcn=sps_rtmsupport('NameChangeFcn',gcbh);  PreCopyFcn=sps_rtmsupport('PreCopyFcn',gcbh);  OpenFcn=sps_rtmsupport('OpenFcn',gcbh, [3 7 8 9]);  CloseFcn=sps_rtmsupport('CloseFcn',gcbh);  PreDeleteFcn=sps_rtmsupport('PreDeleteFcn',gcbh);
      mask Help: helpview(psbhelp);
      mask Callback External: powericon('BreakerCback',gcb);
      mask Callback BreakerResistance: powericon('SwitchesEnables',gcb,'Breaker');
      mask TypeOptions Measurements: None | Branch voltage | Branch current | Branch voltage and current
      mask Display: % plot(X.p1,Y.p1,X.p2,Y.p2,X.p3,Y.p3,X.p4,Y.p4,X.p5,Y.p5,X.p6,Y.p6)
  C4 : Constant  Value=External
  Constant1 : Constant  Value=SwitchA
  Constant2 : Constant  Value=SwitchB
  Constant3 : Constant  Value=SwitchC
  Constant5 : Constant  Value=InitialState
  Stair Generator : powerlib_meascontrol/Pulse & Signal Generators/Stair Generator  t=Switch_Times  e=SwitchStatus  Ts=Ts
      settings: SourceProductName=Simscape Electrical
  Switch : Switch  Threshold=0.5  ZeroCross=off  InputSameDT=on
  Switch1 : Switch  Threshold=0.5  ZeroCross=off  InputSameDT=on
  Switch2 : Switch  Threshold=0.5  ZeroCross=off  InputSameDT=on
  Switch3 : Switch  Threshold=0.5  ZeroCross=off
  ThreePhaseBreaker : PMComponent  PhysicalDomain=powersysdomain  LeftPortType=p1  RightPortType=p1  LConnTagsString=A|B|C  RConnTagsString=a|b|c  mask(InnerPowersysBlock){}
  A : PMIOPort  Side=Left
  B : PMIOPort  Port=2  Side=Left
  C : PMIOPort  Port=3  Side=Left
  a : PMIOPort  Port=4  Side=Right
  b : PMIOPort  Port=5  Side=Right
  c : PMIOPort  Port=6  Side=Right
  wires:
  Constant5/1 -> Switch2/3, Switch1/3, Switch/3
  Stair Generator/1 -> Switch3/3
  com/1 -> Switch3/1
  C4/1 -> Switch3/2
  Switch1/1 -> Breaker B/1(c)
  Constant2/1 -> Switch1/2
  Switch2/1 -> Breaker C/1(c)
  Constant3/1 -> Switch2/2
  Switch/1 -> Breaker A/1(c)
  Constant1/1 -> Switch/2
  Switch3/1 -> Switch/1, Switch1/1, Switch2/1
  connections:
  c/RConn1 -- Breaker C/RConn1 -- ThreePhaseBreaker/LConn3
  b/RConn1 -- Breaker B/RConn1 -- ThreePhaseBreaker/LConn2
  Breaker A/RConn1 -- ThreePhaseBreaker/LConn1 -- a/RConn1
  C/RConn1 -- Breaker C/LConn1 -- ThreePhaseBreaker/RConn3
  B/RConn1 -- Breaker B/LConn1 -- ThreePhaseBreaker/RConn2
  A/RConn1 -- ThreePhaseBreaker/RConn1 -- Breaker A/LConn1

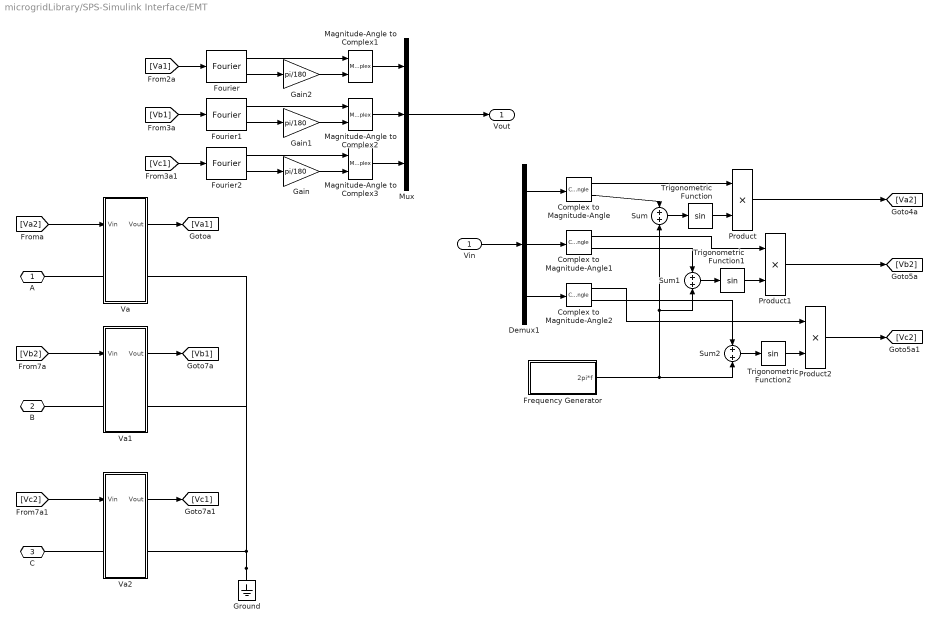
== system microgridLibrary/SPS-Simulink Interface/EMT ==
  Vin : Inport
      settings: SignalType=complex
  Complex to Magnitude-Angle : ComplexToMagnitudeAngle
  Complex to Magnitude-Angle1 : ComplexToMagnitudeAngle
  Complex to Magnitude-Angle2 : ComplexToMagnitudeAngle
  Demux1 : Demux  Outputs=3
  Fourier : powerlib_meascontrol/Measurements/Fourier  Freq=60  n=1  InInit=[1, 0]  Ts=Ts
      settings: SourceProductName=Simscape Electrical
  Fourier1 : powerlib_meascontrol/Measurements/Fourier  Freq=60  n=1  InInit=[1, 0]  Ts=Ts
      settings: SourceProductName=Simscape Electrical
  Fourier2 : powerlib_meascontrol/Measurements/Fourier  Freq=60  n=1  InInit=[1, 0]  Ts=Ts
      settings: SourceProductName=Simscape Electrical
  Frequency Generator : Subsystem  VariantControlMode=Label  Variant=on  LabelModeActiveChoice=Continuous
  Gain : Gain  Gain=pi/180
  Gain1 : Gain  Gain=pi/180
  Gain2 : Gain  Gain=pi/180
  Ground : powerlib/Elements/Ground  LConnTagsString=a
      settings: SourceProductName=Simscape Electrical
  Magnitude-Angle to Complex1 : MagnitudeAngleToComplex
  Magnitude-Angle to Complex2 : MagnitudeAngleToComplex
  Magnitude-Angle to Complex3 : MagnitudeAngleToComplex
  Mux : Mux  Inputs=3
  Product : Product
  Product1 : Product
  Product2 : Product
  Sum : Sum
  Sum1 : Sum
  Sum2 : Sum
  Trigonometric Function : Trigonometry
  Trigonometric Function1 : Trigonometry
  Trigonometric Function2 : Trigonometry
  Va : Subsystem
  Va1 : Subsystem
  Va2 : Subsystem
  A : PMIOPort  Side=Right
  B : PMIOPort  Port=2  Side=Right
  C : PMIOPort  Port=3  Side=Right
  Vout : Outport  VectorParamsAs1DForOutWhenUnconnected=off
      settings: SignalType=complex
  wires:
  Complex to Magnitude-Angle2/2 -> Sum2/1
  Sum2/1 -> Trigonometric Function2/1
  Trigonometric Function2/1 -> Product2/2
  Complex to Magnitude-Angle2/1 -> Product2/1
  Complex to Magnitude-Angle1/1 -> Product1/1
  Trigonometric Function1/1 -> Product1/2
  Sum1/1 -> Trigonometric Function1/1
  Complex to Magnitude-Angle1/2 -> Sum1/1
  Frequency Generator/1(2pi*f) -> Sum/2, Sum1/2, Sum2/2
  Complex to Magnitude-Angle/2 -> Sum/1
  Sum/1 -> Trigonometric Function/1
  Trigonometric Function/1 -> Product/2
  Complex to Magnitude-Angle/1 -> Product/1
  Demux1/3 -> Complex to Magnitude-Angle2/1
  Demux1/2 -> Complex to Magnitude-Angle1/1
  Demux1/1 -> Complex to Magnitude-Angle/1
  Gain2/1 -> Magnitude-Angle to Complex1/2
  Gain1/1 -> Magnitude-Angle to Complex2/2
  Gain/1 -> Magnitude-Angle to Complex3/2
  Magnitude-Angle to Complex2/1 -> Mux/2
  Magnitude-Angle to Complex3/1 -> Mux/3
  Fourier2/2 -> Gain/1
  Fourier2/1 -> Magnitude-Angle to Complex3/1
  Fourier1/2 -> Gain1/1
  Fourier1/1 -> Magnitude-Angle to Complex2/1
  Magnitude-Angle to Complex1/1 -> Mux/1
  Fourier/1 -> Magnitude-Angle to Complex1/1
  Fourier/2 -> Gain2/1
  [Vc1] -> Fourier2/1
  [Vb1] -> Fourier1/1
  [Va1] -> Fourier/1
  Vin/1 -> Demux1/1
  Mux/1 -> Vout/1
  Product/1 -> [Va2]
  Product1/1 -> [Vb2]
  [Va2] -> Va/1(Vin)
  Va/1(Vout) -> [Va1]
  [Vb2] -> Va1/1(Vin)
  Va1/1(Vout) -> [Vb1]
  Va2/1(Vout) -> [Vc1]
  [Vc2] -> Va2/1(Vin)
  Product2/1 -> [Vc2]
  connections:
  Ground/LConn1 -- Va2/RConn1 -- Va1/RConn1 -- Va/RConn1
  Va/LConn1 -- A/RConn1
  Va1/LConn1 -- B/RConn1
  Va2/LConn1 -- C/RConn1

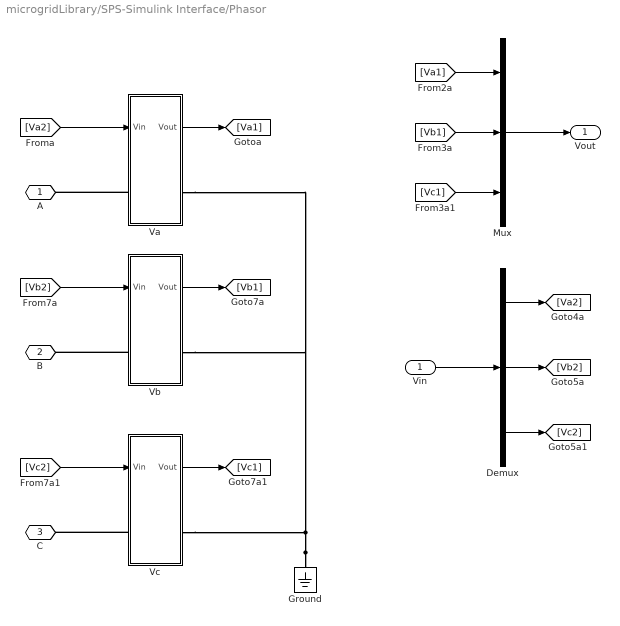
== system microgridLibrary/SPS-Simulink Interface/Phasor ==
  Vin : Inport
  Demux : Demux  Outputs=3
  Ground : powerlib/Elements/Ground  LConnTagsString=a
      settings: SourceProductName=Simscape Electrical
  Mux : Mux  Inputs=3
  Va : Subsystem
  Vb : Subsystem
  Vc : Subsystem
  A : PMIOPort  Side=Right
  B : PMIOPort  Port=2  Side=Right
  C : PMIOPort  Port=3  Side=Right
  Vout : Outport  VectorParamsAs1DForOutWhenUnconnected=off
  wires:
  Vin/1 -> Demux/1
  Mux/1 -> Vout/1
  [Va1] -> Mux/1
  [Vb1] -> Mux/2
  Demux/1 -> [Va2]
  Demux/2 -> [Vb2]
  [Va2] -> Va/1(Vin)
  Va/1(Vout) -> [Va1]
  [Vb2] -> Vb/1(Vin)
  Vb/1(Vout) -> [Vb1]
  Vc/1(Vout) -> [Vc1]
  [Vc2] -> Vc/1(Vin)
  [Vc1] -> Mux/3
  Demux/3 -> [Vc2]
  connections:
  Ground/LConn1 -- Vc/RConn1 -- Vb/RConn1 -- Va/RConn1
  Va/LConn1 -- A/RConn1
  Vb/LConn1 -- B/RConn1
  Vc/LConn1 -- C/RConn1

== system microgridLibrary/Solar Array (EMT Model)/DC Link ==
  C1 : powerlib/Elements/Series RLC Branch  LConnTagsString=__new0  RConnTagsString=__new0  BranchType=C  Resistance=1.0  Inductance=1.0  SetiL0=off  InitialCurrent=0  Capacitance=Clink  Setx0=on  InitialVoltage=Vnom_dc/2  Measurements=None
      settings: SourceProductName=Simscape Electrical
  C2 : powerlib/Elements/Series RLC Branch  LConnTagsString=__new0  RConnTagsString=__new0  BranchType=C  Resistance=1e5  Inductance=1.0  SetiL0=off  InitialCurrent=0  Capacitance=Clink  Setx0=on  InitialVoltage=Vnom_dc/2  Measurements=None
      settings: SourceProductName=Simscape Electrical
  "Vdc " : powerlib/Measurements/Voltage Measurement  Tag=PoWeRsYsTeMmEaSuReMeNt  PhasorSimulation=off  OutputType=Magnitude  PSBequivalent=0
      settings: SourceProductName=Simscape Electrical
  PV+ : PMIOPort  Side=Left
  PV-- : PMIOPort  Port=2  Side=Left
  Inv+ : PMIOPort  Port=3  Side=Right
  N : PMIOPort  Port=4  Side=Right
  Inv-- : PMIOPort  Port=5  Side=Right
  Vdc : Outport  VectorParamsAs1DForOutWhenUnconnected=off
  wires:
  "Vdc "/1 -> Vdc/1
  connections:
  C1/LConn1 -- PV+/RConn1 -- "Vdc "/LConn1 -- Inv+/RConn1
  C2/LConn1 -- N/RConn1 -- C1/RConn1
  "Vdc "/LConn2 -- C2/RConn1 -- PV--/RConn1 -- Inv--/RConn1

== system microgridLibrary/Solar Array (EMT Model)/Grid Inverter ==
  note: Harmonic Filter
  Uref : Inport
  10 kvar : powerlib/Elements/Three-Phase Series RLC Load  LConnTagsString=A|B|C  Configuration=Delta  NominalVoltage=Vnom_sec  Vabc=[1e3 1e3 1e3]  Vabcp=[1e3 1e3 1e3]  NominalFrequency=Fnom  UnbalancedPower=off  ActivePower=Pc  InductivePower=0  CapacitivePower=Qc  Pabc=[10e3 9e3 11e3]  QLabc=[100 90 110]  QCabc=[100 90 110]  Pabcp=[10e3 9e3 11e3]  QLabcp=[100 90 110]  QCabcp=[100 90 110]  Measurements=None  LoadType=constant Z
      settings: SourceProductName=Simscape Electrical
  100 kVA 260V / 25 kV : powerlib/Elements/Three-Phase Transformer (Two Windings)  Winding1Connection=Yg  Winding2Connection=Delta (D1)  CoreType=Three single-phase transformers  SetSaturation=off  Hysteresis=off  DataFile='hysteresis'  SetInitialFlux=off  Measurements=None  UNITS=pu  NominalPower=[Pnom Fnom ]  Winding1=[ Vnom_prim , Rxf/2 , Lxf/2 ]  Winding2=[ Vnom_sec , Rxf/2 , Lxf/2 ]  Rm=200  Lm=200  L0=0.5  Saturation=[ 0,0 ; 0.0024,1.2 ; 1.0,1.52 ]  InitialFluxes=[ 0.8 , -0.8 , 0.7 ]  BreakLoop=off  DiscreteSolver=Trapezoidal iterative  DataType=off  TransfoNumber=0
      settings: SourceProductName=Simscape Electrical
  B1 : powerlib/Measurements/Three-Phase V-I Measurement  VoltageMeasurement=phase-to-ground  SetLabelV=off  LabelV=Vabc_B1  Vpu=off  VpuLL=off  CurrentMeasurement=yes  SetLabelI=off  LabelI=Iabc_B1  Ipu=off  Pbase=100e6  Vbase=500e3  OutputType=Magnitude  PhasorSimulation=off  PSBequivalent=0
      settings: SourceProductName=Simscape Electrical
  Bus Creator : BusCreator  Inputs=2
  Ground : Ground
  L : powerlib/Elements/Three-Phase Series RLC Branch  LConnTagsString=A|B|C  RConnTagsString=A|B|C  BranchType=RL  Resistance=Rchoke*Zbase  Inductance=Lchoke*Zbase/(2*pi*Fnom)  Capacitance=inf  Measurements=None
      settings: SourceProductName=Simscape Electrical
  Three-Level NPC Converter : powerlib/Power Electronics/Three-Level NPC Converter  ModelType=Average model (Uref-controlled)  Ron=1e-3  Rs=1e6  Cs=inf  Vforward=[0,0]  Ron_Diode=1e-3  Rs_Diode=1e6  Cs_Diode=inf  Vf_Diode=1e-3  Rs_CurrentSource=inf
      settings: SourceProductName=Simscape Electrical  SourceProductBaseCode=PS
  Inv+ : PMIOPort  Side=Left
  N : PMIOPort  Port=2  Side=Left
  Inv-- : PMIOPort  Port=3  Side=Left
  A : PMIOPort  Port=4  Side=Right
  B : PMIOPort  Port=5  Side=Right
  C : PMIOPort  Port=6  Side=Right
  m : Outport  VectorParamsAs1DForOutWhenUnconnected=off
  wires:
  Ground/1 -> Three-Level NPC Converter/2
  Bus Creator/1 -> m/1
  B1/2 -> Bus Creator/2  "Iabc"
  B1/1 -> Bus Creator/1  "Vabc"
  Uref/1 -> Three-Level NPC Converter/1
  connections:
  N/RConn1 -- Three-Level NPC Converter/RConn2
  Three-Level NPC Converter/LConn3 -- L/LConn3
  Three-Level NPC Converter/LConn2 -- L/LConn2
  Three-Level NPC Converter/LConn1 -- L/LConn1
  100 kVA 260V / 25 kV/LConn1 -- B1/LConn1
  100 kVA 260V / 25 kV/LConn2 -- B1/LConn2
  100 kVA 260V / 25 kV/LConn3 -- B1/LConn3
  10 kvar/LConn2 -- 100 kVA 260V / 25 kV/RConn2 -- L/RConn2
  10 kvar/LConn3 -- 100 kVA 260V / 25 kV/RConn3 -- L/RConn3
  Three-Level NPC Converter/RConn3 -- Inv--/RConn1
  Three-Level NPC Converter/RConn1 -- Inv+/RConn1
  L/RConn1 -- 100 kVA 260V / 25 kV/RConn1 -- 10 kvar/LConn1
  B1/RConn1 -- A/RConn1
  B1/RConn2 -- B/RConn1
  B1/RConn3 -- C/RConn1
